simulink model "Environment_test"  (R2019a)
settings: Solver=VariableStepAuto  StartTime=0.0  StopTime=10.0  RelTol=1e-3
values from neighbouring files (symbols this model uses):
  JD = jday(Yr,Month,Day,Hr,Min,Sec)    [sgp4_test.m]
settings Model: Creator=mario  LastModifiedBy=mario

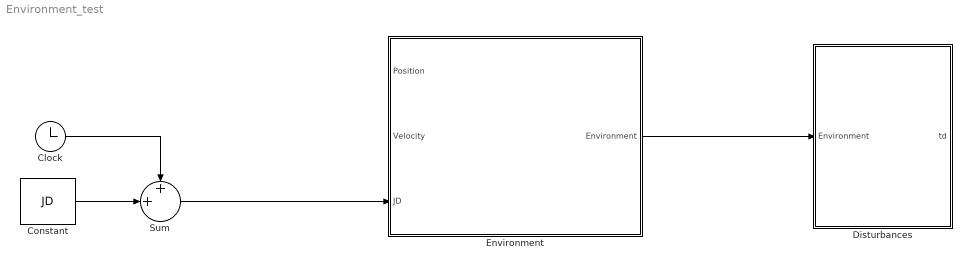
== system Environment_test ==
  Clock : Clock
  Constant : Constant  Value=JD
  Disturbances : Subsystem
  Environment : Subsystem
  Sum : Sum  Inputs=++|
  wires:
  Environment/1(Environment) -> Disturbances/1(Environment)
  Constant/1 -> Sum/2
  Clock/1 -> Sum/1
  Sum/1 -> Environment/3(JD)

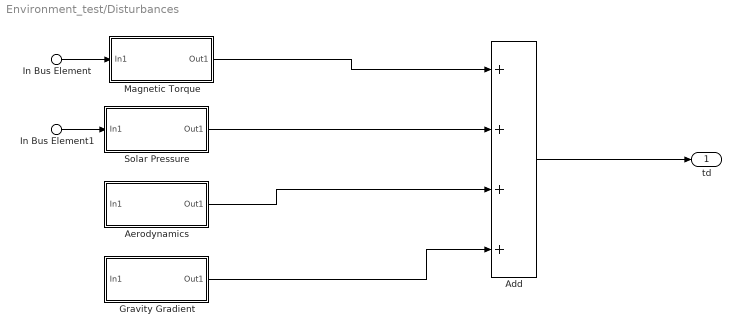
== system Environment_test/Disturbances ==
  In Bus Element : Inport  PortName=Environment  Element=Mag_vector
  In Bus Element1 : Inport  PortName=Environment  Element=Sun_vector
  Add : Sum  Inputs=4
  Aerodynamics : Subsystem
  Gravity Gradient : Subsystem
  Magnetic Torque : Subsystem
  Solar Pressure : Subsystem
  td : Outport
  wires:
  Add/1 -> td/1
  Magnetic Torque/1(Out1) -> Add/1
  Solar Pressure/1(Out1) -> Add/2
  Aerodynamics/1(Out1) -> Add/3
  Gravity Gradient/1(Out1) -> Add/4
  In Bus Element/1 -> Magnetic Torque/1(In1)
  In Bus Element1/1 -> Solar Pressure/1(In1)

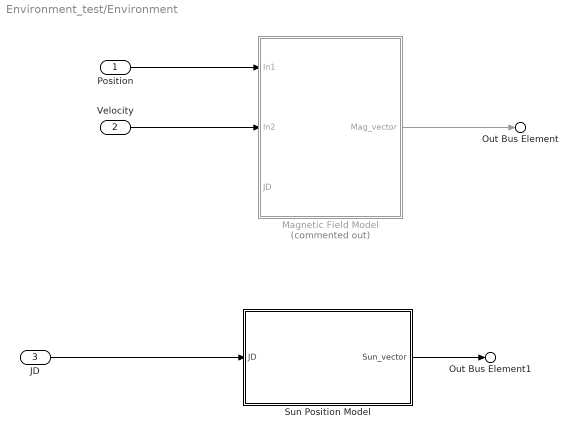
== system Environment_test/Environment ==
  Position : Inport
  Velocity : Inport  Port=2
  JD : Inport  Port=3
  Magnetic Field Model : Subsystem  Commented=on
  Sun Position Model : Subsystem
  Out Bus Element : Outport  PortName=Environment  Element=Mag_vector
  Out Bus Element1 : Outport  PortName=Environment  Element=Sun_vector
  wires:
  Position/1 -> Magnetic Field Model/1(In1)
  Velocity/1 -> Magnetic Field Model/2(In2)
  Sun Position Model/1(Sun_vector) -> Out Bus Element1/1
  Magnetic Field Model/1(Mag_vector) -> Out Bus Element/1
  JD/1 -> Sun Position Model/1(JD)

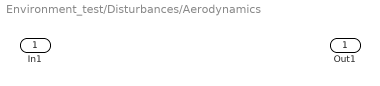
== system Environment_test/Disturbances/Aerodynamics ==
  In1 : Inport
  Out1 : Outport

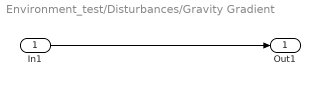
== system Environment_test/Disturbances/Gravity Gradient ==
  In1 : Inport
  Out1 : Outport
  wires:
  In1/1 -> Out1/1

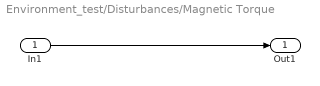
== system Environment_test/Disturbances/Magnetic Torque ==
  In1 : Inport
  Out1 : Outport
  wires:
  In1/1 -> Out1/1

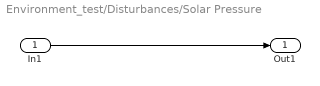
== system Environment_test/Disturbances/Solar Pressure ==
  In1 : Inport
  Out1 : Outport
  wires:
  In1/1 -> Out1/1

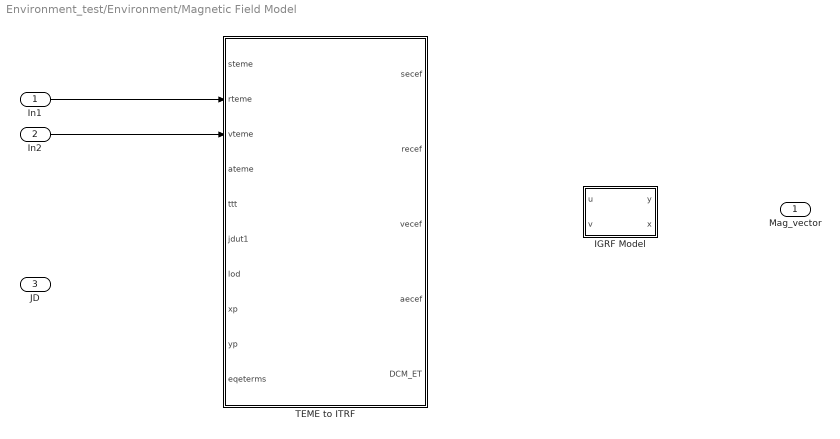
== system Environment_test/Environment/Magnetic Field Model ==
  In1 : Inport
  In2 : Inport  Port=2
  JD : Inport  Port=3
  IGRF Model : MATLAB Function  TreatAsAtomicUnit=on
  TEME to ITRF : MATLAB Function  TreatAsAtomicUnit=on
  Mag_vector : Outport  VectorParamsAs1DForOutWhenUnconnected=on
  wires:
  In1/1 -> TEME to ITRF/2(rteme)
  In2/1 -> TEME to ITRF/3(vteme)

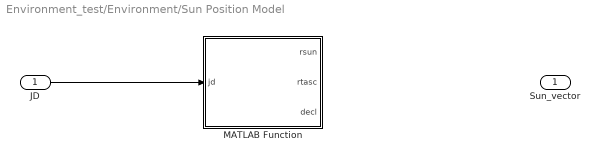
== system Environment_test/Environment/Sun Position Model ==
  JD : Inport
  MATLAB Function : MATLAB Function  TreatAsAtomicUnit=on
  Sun_vector : Outport  VectorParamsAs1DForOutWhenUnconnected=on
  wires:
  JD/1 -> MATLAB Function/1(jd)

== matlab function Environment_test/Environment/Magnetic Field Model/TEME to ITRF ==
  data: steme input; secef output; rteme input; recef output; vteme input; ateme input; ttt input; jdut1 input; lod input; xp input; yp input; eqeterms input; vecef output; aecef output; DCM_ET output
% ----------------------------------------------------------------------------
%
%                           function teme2ecef
%
%  this function trsnforms a vector from the true equator mean equniox frame
%    (teme), to an earth fixed (ITRF) frame.  the results take into account
%    the effects of sidereal time, and polar motion.
%
%  author        : david vallado                  719-573-2600   30 oct 2017
%
%  revisions
%
%  inputs          description                    range / units
%    rteme       - position vector teme           km
%    steme       - another position vector teme   km
%    vteme       - velocity vector teme           km/s
%    ateme       - acceleration vector teme       km/s2
%    ttt         - julian centuries of tt         centuries
%    jdut1       - julian date of ut1             days from 4713 bc
%    lod         - excess length of day           sec
%    xp          - polar motion coefficient       rad
%    yp          - polar motion coefficient       rad
%    eqeterms    - use extra two terms (kinematic) after 1997  0, 2
%
%  outputs       :
%    recef       - position vector earth fixed    km
%    secef       - another position vector earth fixed    km
%    vecef       - velocity vector earth fixed    km/s
%    aecef       - acceleration vector earth fixedkm/s2
%
%  locals        :
%    st          - matrix for pef - tod 
%    pm          - matrix for ecef - pef 
%
%  coupling      :
%   gstime       - greenwich mean sidereal time   rad
%   polarm       - rotation for polar motion      pef - ecef
%
%  references    :
%    vallado       2013, 231-233
%
% [recef, vecef, aecef] = teme2ecef( rteme, vteme, ateme, ttt, jdut1, lod, xp, yp, eqeterms );
% ----------------------------------------------------------------------------

function [secef, recef, vecef, aecef, DCM_ET] = teme2ecef(steme, rteme, vteme, ateme, ttt, jdut1, lod, xp, yp, eqeterms )

        deg2rad = pi/180.0;
        
        
        % ------------------------ find gmst --------------------------
        gmst= gstime( jdut1 );

        % find omega from nutation theory
        omega=  125.04452222  + (   -6962890.5390 *ttt + ...
                7.455 *ttt*ttt + 0.008 *ttt*ttt*ttt )  / 3600.0;
        omega= rem( omega, 360.0  ) * deg2rad;
        
        % ------------------------ find mean ast ----------------------
        % teme does not include the geometric terms here
        % after 1997, kinematic terms apply
        if (jdut1 > 2450449.5 ) && (eqeterms > 0)
            gmstg = gmst ...
                   + 0.00264*pi /(3600*180)*sin(omega) ...
                   + 0.000063*pi /(3600*180)*sin(2.0 *omega);
        else
            gmstg = gmst;
        end

        gmstg = rem (gmstg, 2.0*pi);

        st = zeros(3,3);
        st(1,1) =  cos(gmstg);
        st(1,2) = -sin(gmstg);
        st(1,3) =  0.0;
        st(2,1) =  sin(gmstg);
        st(2,2) =  cos(gmstg);
        st(2,3) =  0.0;
        st(3,1) =  0.0;
        st(3,2) =  0.0;
        st(3,3) =  1.0;

        [pm] = polarm(xp,yp,ttt,'80');

        rpef  = st'*rteme;
        recef = pm'*rpef;
 
        spef  = st'*steme;
        secef = pm'*spef;

        thetasa    = 7.29211514670698e-05 * (1.0  - lod/86400.0 );
        omegaearth = [0; 0; thetasa;];

        vpef  = st'*vteme - cross( omegaearth,rpef );
        vecef = pm'*vpef;

        temp  = cross(omegaearth,rpef);

        aecef = pm'*(st'*ateme - cross(omegaearth,temp) ...
                - 2.0*cross(omegaearth,vpef));
        DCM_ET = pm'*st;

%fprintf(1,'st gmst %11.8f ast %11.8f ome  %11.8f \n', gmst*180/pi, ast*180/pi, omegaearth*180/pi );
% -----------------------------------------------------------------------------
%
%                           function gstime
%
%  this function finds the greenwich sidereal time (iau-82).
%
%  author        : david vallado                  719-573-2600    7 jun 2002
%
%  revisions
%                -
%
%  inputs          description                    range / units
%    jdut1       - julian date of ut1             days from 4713 bc
%
%  outputs       :
%    gst         - greenwich sidereal time        0 to 2pi rad
%
%  locals        :
%    temp        - temporary variable for reals   rad
%    tut1        - julian centuries from the
%                  jan 1, 2000 12 h epoch (ut1)
%
%  coupling      :
%
%  references    :
%    vallado       2007, 193, Eq 3-43
%
% gst = gstime(jdut1);
% -----------------------------------------------------------------------------

function gst = gstime(jdut1)

        twopi      = 2.0*pi;
        deg2rad    = pi/180.0;

        % ------------------------  implementation   ------------------
        tut1= ( jdut1 - 2451545.0 ) / 36525.0;

        temp = - 6.2e-6 * tut1 * tut1 * tut1 + 0.093104 * tut1 * tut1  ...
               + (876600.0 * 3600.0 + 8640184.812866) * tut1 + 67310.54841;

        % 360/86400 = 1/240, to deg, to rad
        temp = rem( temp*deg2rad/240.0,twopi );

        % ------------------------ check quadrants --------------------
        if ( temp < 0.0 )
            temp = temp + twopi;
        end

        gst = temp;

%?
% ----------------------------------------------------------------------------
%
%                           function polarm
%
%  this function calulates the transformation matrix that accounts for polar
%    motion. both the 1980 and 2000 theories are handled. note that the rotation 
%    order is different between 1980 and 2000 .
%
%  author        : david vallado                  719-573-2600   25 jun 2002
%
%  revisions
%    vallado     - consolidate with iau 2000                     14 feb 2005
%
%  inputs          description                    range / units
%    xp          - polar motion coefficient       rad
%    yp          - polar motion coefficient       rad
%    ttt         - julian centuries of tt (00 theory only)
%    opt         - method option                  '01', '02', '80'
%
%  outputs       :
%    pm          - transformation matrix for ecef - pef
%
%  locals        :
%    convrt      - conversion from arcsec to rad
%    sp          - s prime value
%
%  coupling      :
%    none.
%
%  references    :
%    vallado       2004, 207-209, 211, 223-224
%
% [pm] = polarm ( xp, yp, ttt, opt );
% ----------------------------------------------------------------------------

function [pm] = polarm ( xp, yp, ttt, opt )


        cosxp = cos(xp);
        sinxp = sin(xp);
        cosyp = cos(yp);
        sinyp = sin(yp);

        if (opt == '80')
            pm = zeros(3,3);
            pm(1,1) =  cosxp;
            pm(1,2) =  0.0;
            pm(1,3) = -sinxp;
            pm(2,1) =  sinxp * sinyp;
            pm(2,2) =  cosyp;
            pm(2,3) =  cosxp * sinyp;
            pm(3,1) =  sinxp * cosyp;
            pm(3,2) = -sinyp;
            pm(3,3) =  cosxp * cosyp;

            % a1 = rot2mat(xp);
            % a2 = rot1mat(yp);
            % pm = a2*a1;          
            % Approximate matrix using small angle approximations
            %pm(1,1) =  1.0;
            %pm(2,1) =  0.0;
            %pm(3,1) =  xp;
            %pm(1,2) =  0.0;
            %pm(2,2) =  1.0;
            %pm(3,2) = -yp;
            %pm(1,3) = -xp;
            %pm(2,3) =  yp;
            %pm(3,3) =  1.0;
        else  
            convrt = pi / (3600.0*180.0);
            % approximate sp value in rad
            sp = -47.0e-6 * ttt * convrt;
            cossp = cos(sp);
            sinsp = sin(sp);

            % form the matrix
            pm = zeros(3,3);
            pm(1,1) =  cosxp * cossp;
            pm(1,2) = -cosyp * sinsp + sinyp * sinxp * cossp;
            pm(1,3) = -sinyp * sinsp - cosyp * sinxp * cossp;
            pm(2,1) =  cosxp * sinsp;
            pm(2,2) =  cosyp * cossp + sinyp * sinxp * sinsp;
            pm(2,3) =  sinyp * cossp - cosyp * sinxp * sinsp;
            pm(3,1) =  sinxp;
            pm(3,2) = -sinyp * cosxp;
            pm(3,3) =  cosyp * cosxp;

            % a1 = rot1mat(yp);
            % a2 = rot2mat(xp);
            % a3 = rot3mat(-sp);
            % pm = a3*a2*a1;
        end

== matlab function Environment_test/Environment/Magnetic Field Model/IGRF Model ==
  data: u input; y output; v input; x output
function [y,x] = fcn(u,v)

y = u;
x = v;

== matlab function Environment_test/Environment/Sun Position Model/MATLAB Function ==
  data: jd input; rsun output; rtasc output; decl output
% ------------------------------------------------------------------------------
%
%                           function sun
%
%  this function calculates the geocentric equatorial position vector
%    the sun given the julian date.  this is the low precision formula and
%    is valid for years from 1950 to 2050.  accuaracy of apparent coordinates
%    is 0.01  degrees.  notice many of the calculations are performed in
%    degrees, and are not changed until later.  this is due to the fact that
%    the almanac uses degrees exclusively in their formulations.
%
%  author        : david vallado                  719-573-2600   27 may 2002
%
%  revisions
%    vallado     - fix mean lon of sun                            7 mat 2004
%
%  inputs          description                    range / units
%    jd          - julian date                    days from 4713 bc
%
%  outputs       :
%    rsun        - ijk position vector of the sun au
%    rtasc       - right ascension                rad
%    decl        - declination                    rad
%
%  locals        :
%    meanlong    - mean longitude
%    meananomaly - mean anomaly
%    eclplong    - ecliptic longitude
%    obliquity   - mean obliquity of the ecliptic
%    tut1        - julian centuries of ut1 from
%                  jan 1, 2000 12h
%    ttdb        - julian centuries of tdb from
%                  jan 1, 2000 12h
%    hr          - hours                          0 .. 24              10
%    min         - minutes                        0 .. 59              15
%    sec         - seconds                        0.0  .. 59.99          30.00
%    temp        - temporary variable
%    deg         - degrees
%
%  coupling      :
%    none.
%
%  references    :
%    vallado       2007, 281, alg 29, ex 5-1
%
% [rsun,rtasc,decl] = sun ( jd );
% ------------------------------------------------------------------------------

function [rsun,rtasc,decl] = sun ( jd )

        twopi      =     2.0*pi;
        deg2rad    =     pi/180.0;
        show = 'n';
        rsun = zeros(3,1);
        
        % -------------------------  implementation   -----------------
        % -------------------  initialize values   --------------------
        tut1= ( jd - 2451545.0  )/ 36525.0;

        if show == 'y'
            fprintf(1,'tut1 %14.9f \n',tut1);
        end

        meanlong= 280.460  + 36000.77*tut1;
        meanlong= rem( meanlong,360.0  );  %deg

        ttdb= tut1;
        meananomaly= 357.5277233  + 35999.05034 *ttdb;
        meananomaly= rem( meananomaly*deg2rad,twopi );  %rad
        if ( meananomaly < 0.0  )
            meananomaly= twopi + meananomaly;
        end

        eclplong= meanlong + 1.914666471 *sin(meananomaly) ...
                    + 0.019994643 *sin(2.0 *meananomaly); %deg
        eclplong= rem( eclplong,360.0  );  %deg

        obliquity= 23.439291  - 0.0130042 *ttdb;  %deg

        eclplong = eclplong *deg2rad;
        obliquity= obliquity *deg2rad;

        % --------- find magnitude of sun vector, )   components ------
        magr= 1.000140612  - 0.016708617 *cos( meananomaly ) ...
                              - 0.000139589 *cos( 2.0 *meananomaly );    % in au's

        rsun(1)= magr*cos( eclplong );
        rsun(2)= magr*cos(obliquity)*sin(eclplong);
        rsun(3)= magr*sin(obliquity)*sin(eclplong);

        if show == 'y'
            fprintf(1,'meanlon %11.6f meanan %11.6f eclplon %11.6f obli %11.6f \n', ...
                    meanlong,meananomaly/deg2rad,eclplong/deg2rad,obliquity/deg2rad);
            fprintf(1,'rs %11.9f %11.9f %11.9f \n',rsun);
            fprintf(1,'magr %14.7f \n',magr);
        end

        rtasc= atan( cos(obliquity)*tan(eclplong) );

        % --- check that rtasc is in the same quadrant as eclplong ----
        if ( eclplong < 0.0  )
            eclplong= eclplong + twopi;    % make sure it's in 0 to 2pi range
        end
        if ( abs( eclplong-rtasc ) > pi*0.5  )
            rtasc= rtasc + 0.5 *pi*round( (eclplong-rtasc)/(0.5 *pi));
        end
        decl = asin( sin(obliquity)*sin(eclplong) );
